simulink model "keyEventCombiner"  (R2016b)
settings: Solver=VariableStepAuto  StartTime=0.0  StopTime=10.0  RelTol=1e-3
settings Model: DataDictionary=DataDictionary.sldd  Creator=Taeke  LastModifiedBy=Taeke

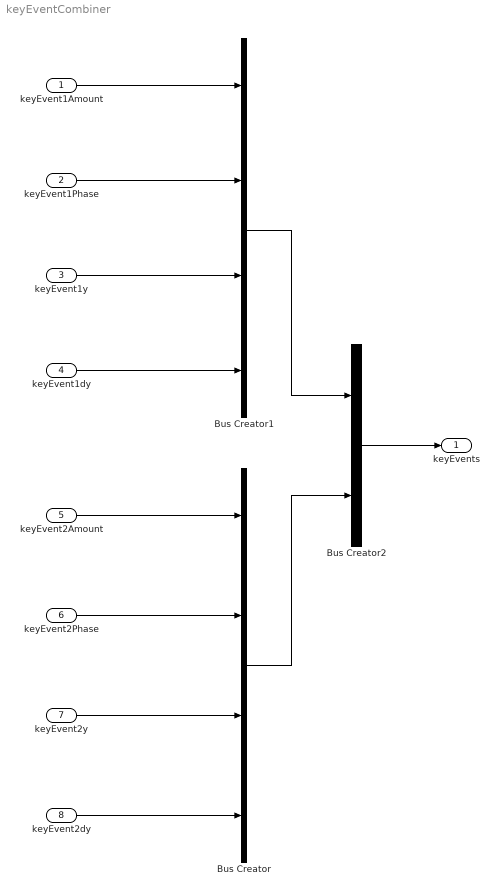
== system keyEventCombiner ==
  keyEvent1Amount : Inport
  keyEvent1Phase : Inport  Port=2
  keyEvent1y : Inport  Port=3
  keyEvent1dy : Inport  Port=4
  keyEvent2Amount : Inport  Port=5
  keyEvent2Phase : Inport  Port=6
  keyEvent2y : Inport  Port=7
  keyEvent2dy : Inport  Port=8
  Bus Creator : BusCreator  Inputs=4
  Bus Creator1 : BusCreator  Inputs=4
  Bus Creator2 : BusCreator  Inputs=2
  keyEvents : Outport  OutDataTypeStr=Bus: keyEventTotal
  wires:
  keyEvent2Amount/1 -> Bus Creator/1
  keyEvent2dy/1 -> Bus Creator/4
  keyEvent2y/1 -> Bus Creator/3
  keyEvent2Phase/1 -> Bus Creator/2
  keyEvent1Amount/1 -> Bus Creator1/1
  keyEvent1y/1 -> Bus Creator1/3
  keyEvent1dy/1 -> Bus Creator1/4
  keyEvent1Phase/1 -> Bus Creator1/2
  Bus Creator1/1 -> Bus Creator2/1
  Bus Creator/1 -> Bus Creator2/2
  Bus Creator2/1 -> keyEvents/1
